simulink model "Seven_segments"  (R2016b)
settings: Solver=VariableStepAuto  StartTime=0.0  StopTime=10  RelTol=1e-3
settings Model: Creator=rcostado  LastModifiedBy=rcostado

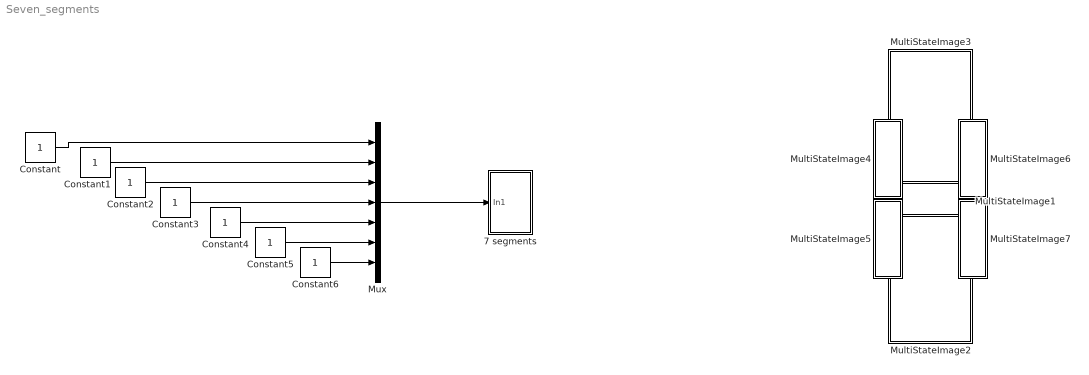
== system Seven_segments ==
  7 segments : Subsystem
  Constant{,1..6} (7 alike) : Constant  OutDataTypeStr=boolean
  MultiStateImage1 : Subsystem  DialogController=hmiCreateDDGDialog  IsWebBlock=on  mask(MWDashboardBlock){webBlockId=e720484e-4967-4559-9ba2-4014e9d9ccbd, webBlockType=multistateimage, ShowInLibBrowser=on, ShowInitialText=on, HMISrcModelName=Seven_segments}
      mask prompts: webBlockType "WebBlock Type"; HMISrcModelName "Source Model"
      mask help: SimulinkHMI:dialogs:MultiStateImageDialogDesc
      mask Help: helpview([docroot '/mapfiles/simulink.map'], 'hmi_multistateimage')
      mask Display:
      | if strcmp(get_param(bdroot(gcb),'BlockDiagramType'), 'library')
      |     image([(matlabroot) '/toolbox/simulink/hmi/icons/MultiStateImage.png']);
      | end
  MultiStateImage2 : Subsystem  DialogController=hmiCreateDDGDialog  IsWebBlock=on  mask(MWDashboardBlock){webBlockId=34e36798-be14-4a4f-ab26-c65eb5c11d48, webBlockType=multistateimage, ShowInLibBrowser=on, ShowInitialText=on, HMISrcModelName=Seven_segments}
      mask prompts: webBlockType "WebBlock Type"; HMISrcModelName "Source Model"
      mask help: SimulinkHMI:dialogs:MultiStateImageDialogDesc
      mask Help: helpview([docroot '/mapfiles/simulink.map'], 'hmi_multistateimage')
      mask Display:
      | if strcmp(get_param(bdroot(gcb),'BlockDiagramType'), 'library')
      |     image([(matlabroot) '/toolbox/simulink/hmi/icons/MultiStateImage.png']);
      | end
  MultiStateImage3 : Subsystem  DialogController=hmiCreateDDGDialog  IsWebBlock=on  mask(MWDashboardBlock){webBlockId=d6091914-40ba-46a9-9a59-a105626dec83, webBlockType=multistateimage, ShowInLibBrowser=on, ShowInitialText=on, HMISrcModelName=Seven_segments}
      mask prompts: webBlockType "WebBlock Type"; HMISrcModelName "Source Model"
      mask help: SimulinkHMI:dialogs:MultiStateImageDialogDesc
      mask Help: helpview([docroot '/mapfiles/simulink.map'], 'hmi_multistateimage')
      mask Display:
      | if strcmp(get_param(bdroot(gcb),'BlockDiagramType'), 'library')
      |     image([(matlabroot) '/toolbox/simulink/hmi/icons/MultiStateImage.png']);
      | end
  MultiStateImage4 : Subsystem  DialogController=hmiCreateDDGDialog  IsWebBlock=on  mask(MWDashboardBlock){webBlockId=1d783cd4-5519-44cd-b15f-7396be9e0a29, webBlockType=multistateimage, ShowInLibBrowser=on, ShowInitialText=on, HMISrcModelName=Seven_segments}
      mask prompts: webBlockType "WebBlock Type"; HMISrcModelName "Source Model"
      mask help: SimulinkHMI:dialogs:MultiStateImageDialogDesc
      mask Help: helpview([docroot '/mapfiles/simulink.map'], 'hmi_multistateimage')
      mask Display:
      | if strcmp(get_param(bdroot(gcb),'BlockDiagramType'), 'library')
      |     image([(matlabroot) '/toolbox/simulink/hmi/icons/MultiStateImage.png']);
      | end
  MultiStateImage5 : Subsystem  DialogController=hmiCreateDDGDialog  IsWebBlock=on  mask(MWDashboardBlock){webBlockId=8518a746-01c5-481b-ab49-a93bebbbf341, webBlockType=multistateimage, ShowInLibBrowser=on, ShowInitialText=on, HMISrcModelName=Seven_segments}
      mask prompts: webBlockType "WebBlock Type"; HMISrcModelName "Source Model"
      mask help: SimulinkHMI:dialogs:MultiStateImageDialogDesc
      mask Help: helpview([docroot '/mapfiles/simulink.map'], 'hmi_multistateimage')
      mask Display:
      | if strcmp(get_param(bdroot(gcb),'BlockDiagramType'), 'library')
      |     image([(matlabroot) '/toolbox/simulink/hmi/icons/MultiStateImage.png']);
      | end
  MultiStateImage6 : Subsystem  DialogController=hmiCreateDDGDialog  IsWebBlock=on  mask(MWDashboardBlock){webBlockId=a751ca72-7e77-4dc2-83f5-e8826a5eaee6, webBlockType=multistateimage, ShowInLibBrowser=on, ShowInitialText=on, HMISrcModelName=Seven_segments}
      mask prompts: webBlockType "WebBlock Type"; HMISrcModelName "Source Model"
      mask help: SimulinkHMI:dialogs:MultiStateImageDialogDesc
      mask Help: helpview([docroot '/mapfiles/simulink.map'], 'hmi_multistateimage')
      mask Display:
      | if strcmp(get_param(bdroot(gcb),'BlockDiagramType'), 'library')
      |     image([(matlabroot) '/toolbox/simulink/hmi/icons/MultiStateImage.png']);
      | end
  MultiStateImage7 : Subsystem  DialogController=hmiCreateDDGDialog  IsWebBlock=on  mask(MWDashboardBlock){webBlockId=7313ed0c-18ea-4374-9166-c592982af777, webBlockType=multistateimage, ShowInLibBrowser=on, ShowInitialText=on, HMISrcModelName=Seven_segments}
      mask prompts: webBlockType "WebBlock Type"; HMISrcModelName "Source Model"
      mask help: SimulinkHMI:dialogs:MultiStateImageDialogDesc
      mask Help: helpview([docroot '/mapfiles/simulink.map'], 'hmi_multistateimage')
      mask Display:
      | if strcmp(get_param(bdroot(gcb),'BlockDiagramType'), 'library')
      |     image([(matlabroot) '/toolbox/simulink/hmi/icons/MultiStateImage.png']);
      | end
  Mux : Mux  Inputs=7
  wires:
  Constant6/1 -> Mux/7
  Constant5/1 -> Mux/6
  Constant4/1 -> Mux/5
  Constant3/1 -> Mux/4
  Constant2/1 -> Mux/3
  Constant1/1 -> Mux/2
  Constant/1 -> Mux/1
  Mux/1 -> 7 segments/1(In1)

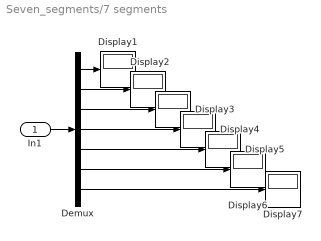
== system Seven_segments/7 segments ==
  In1 : Inport
  Demux : Demux  Outputs=7
  Display{1..7} (7 alike) : Display
  wires:
  Demux/1 -> Display1/1
  Demux/2 -> Display2/1
  Demux/3 -> Display3/1
  Demux/4 -> Display4/1
  Demux/5 -> Display5/1
  Demux/6 -> Display6/1
  Demux/7 -> Display7/1
  In1/1 -> Demux/1

== system Seven_segments/MultiStateImage1 ==

== system Seven_segments/MultiStateImage2 ==

== system Seven_segments/MultiStateImage3 ==

== system Seven_segments/MultiStateImage4 ==

== system Seven_segments/MultiStateImage5 ==

== system Seven_segments/MultiStateImage6 ==

== system Seven_segments/MultiStateImage7 ==
